simulink model "sl_groundvehicleDynamics_test"  (R2025b)
settings: Solver=ode45  StartTime=0.0  StopTime=2000  RelTol=1e-5  EnableMultiTasking=on
InitFcn:
  | mdl_robot;
values from neighbouring files (symbols this model uses):
  optimized_waypoints = two_opt_nn_multi_optimisation(waypoints)    [mdl_robot.m]
  scanAngles = linspace(-fov_half,fov_half, 30)    [param.m]
undefined symbols (not defined in the file or in its folder): obstacles, robot
libraries: mobileRoboticsLib x4, simulink x4, simulink_extras x2, sharedTrackingLibrary x1
(part 2 of 2)

== matlab function sl_groundvehicleDynamics_test/MATLAB Function3 ==
  data: slam_map input; local_cost_map output; pose input; ranges input; scan_angles input; waypoints input; show_map input
function local_cost_map = local_costmap(slam_map, pose, ranges, scan_angles, waypoints, show_map)
% LOCAL_COSTMAP - Creates a local costmap with obstacle avoidance and waypoint attraction
% Inputs:
%   slam_map     - Binary occupancy grid (82x104, 0=free, 1=occupied)
%   pose         - Robot pose [x, y, theta] in meters, radians
%   ranges       - Lidar ranges (meters)
%   scan_angles  - Lidar scan angles (radians)
%   waypoints    - Nx2 matrix of [x, y] target points in meters
%   show_map     - Boolean flag to visualize local costmap
% Output:
%   local_cost_map - Local costmap (0=free, 100=obstacle, attraction=negative cost)

% Parameters
map_size = [52, 41]; % Full map size [m] [x, y]
res = 0.5; % m/cell
rows = round(map_size(2)/res); % 82 rows
cols = round(map_size(1)/res); % 104 cols
window_size = 10; % Local window size [m] (10x10m)
window_cells = round(window_size/res); % e.g., 20 cells
inflation_radius = 0.5; % Buffer for local avoidance
max_cost = 100; % Lethal obstacle cost
inflation_decay = 0.1; % Exponential decay rate
k_att = 20; % attraction gain (tunable)

% Validate inputs
if ~isequal(size(slam_map), [rows, cols])
    error('SLAM map must be %dx%d', rows, cols);
end
if ~isequal(size(pose), [3, 1]) && ~isequal(size(pose), [1, 3])
    error('Pose must be [x, y, theta]');
end
if length(ranges) ~= length(scan_angles)
    error('Ranges and scan_angles must have same length');
end

% Initialize local costmap
local_rows = window_cells;
local_cols = window_cells;
local_cost_map = zeros(local_rows, local_cols);

% Convert robot pose to global grid indices
global_rows = round(map_size(2)/res);
global_cols = round(map_size(1)/res);
robot_row = round(pose(2)/res) + 1;
robot_col = round(pose(1)/res) + 1;

% Extract window from SLAM map
half_window = window_cells/2;
row_start = max(1, robot_row - half_window + 1);
row_end = min(global_rows, robot_row + half_window);
col_start = max(1, robot_col - half_window + 1);
col_end = min(global_cols, robot_col + half_window);

local_row_start = max(1, half_window - (robot_row - 1));
local_row_end = local_row_start + (row_end - row_start);
local_col_start = max(1, half_window - (robot_col - 1));
local_col_end = local_col_start + (col_end - col_start);

local_cost_map(local_row_start:local_row_end, local_col_start:local_col_end) = ...
    slam_map(row_start:row_end, col_start:col_end) * max_cost;

% Insert live lidar data
for i = 1:length(ranges)
    if ranges(i) > 0 && ranges(i) < window_size/2
        end_x = pose(1) + ranges(i) * cos(pose(3) + scan_angles(i));
        end_y = pose(2) + ranges(i) * sin(pose(3) + scan_angles(i));
        [end_row, end_col] = world2grid(end_x, end_y, res, window_size, pose);
        if end_row >= 1 && end_row <= local_rows && end_col >= 1 && end_col <= local_cols
            local_cost_map(end_row, end_col) = max_cost;
        end
    end
end

% Apply inflation
for r = 1:local_rows
    for c = 1:local_cols
        if local_cost_map(r, c) == max_cost
            continue;
        end
        min_dist = inf;
        for r2 = 1:local_rows
            for c2 = 1:local_cols
                if local_cost_map(r2, c2) == max_cost
                    world_dist = res * norm([r-r2, c-c2]);
                    min_dist = min(min_dist, world_dist);
                end
            end
        end
        if min_dist <= inflation_radius
            local_cost_map(r, c) = max_cost * exp(-inflation_decay * min_dist);
        end
    end
end

% --- Waypoint Attraction (negative costs) ---
for wp = 1:size(waypoints,1)
    wp_x = waypoints(wp,1);
    wp_y = waypoints(wp,2);
    [wp_row, wp_col] = world2grid(wp_x, wp_y, res, window_size, pose);
    if wp_row>=1 && wp_row<=local_rows && wp_col>=1 && wp_col<=local_cols
        for r = 1:local_rows
            for c = 1:local_cols
                dist = res * norm([r-wp_row, c-wp_col]);
                local_cost_map(r,c) = local_cost_map(r,c) - k_att * exp(-0.5*dist); 
            end
        end
    end
end

% Normalize: clamp costs
local_cost_map(local_cost_map > max_cost) = max_cost;
local_cost_map(local_cost_map < -max_cost/2) = -max_cost/2; % attraction cap

% Ensure free space baseline is 0 or negative (for attraction)
local_cost_map(local_cost_map < 1 & local_cost_map > -1) = 0;

% Visualization
if show_map
    figure(4);
    imagesc([-window_size/2, window_size/2], [-window_size/2, window_size/2], local_cost_map);
    colormap(jet); % now negative = blue, positive = red
    set(gca, 'YDir', 'normal');
    axis equal tight;
    xlabel('X [m]'); ylabel('Y [m]');
    title('Local Costmap with Obstacles and Waypoint Attraction');
    colorbar;
    hold on;
    % robot pose
    plot(0, 0, 'ro', 'MarkerSize', 8, 'LineWidth', 2);
    x_end = 0.5*cos(pose(3)); y_end = 0.5*sin(pose(3));
    plot([0, x_end], [0, y_end], 'r-', 'LineWidth', 2);
    % waypoints
    for wp = 1:size(waypoints,1)
        wx = waypoints(wp,1) - pose(1);
        wy = waypoints(wp,2) - pose(2);
        plot(wx, wy, 'gx', 'MarkerSize', 10, 'LineWidth', 2);
    end
    hold off;
end

end

% Helper: Convert world to local grid indices
function [row, col] = world2grid(x, y, res, window_size, robot_pose)
    x_local = x - robot_pose(1) + window_size/2;
    y_local = y - robot_pose(2) + window_size/2;
    col = round(x_local / res) + 1;
    row = round(y_local / res) + 1;
end
